simulink model "forcesimulationmodel"  (R2023a)
settings: Solver=VariableStepAuto  StartTime=0.0  StopTime=0.06  RelTol=1e-3
undefined symbols (not defined in the file): tstep
settings Model: Creator=s202421  LastModifiedBy=s202421

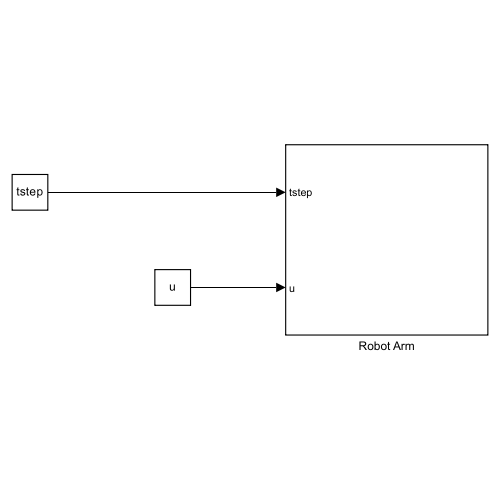
[thumbnail: Simulink's stored preview of the top-level diagram]
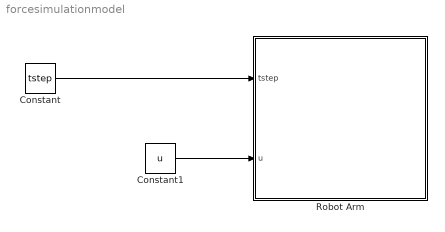
== system forcesimulationmodel ==
  Constant : Constant  Value=tstep
  Constant1 : Constant  Value=u
  Robot Arm : Subsystem
  wires:
  Constant/1 -> Robot Arm/1(tstep)
  Constant1/1 -> Robot Arm/2(u)

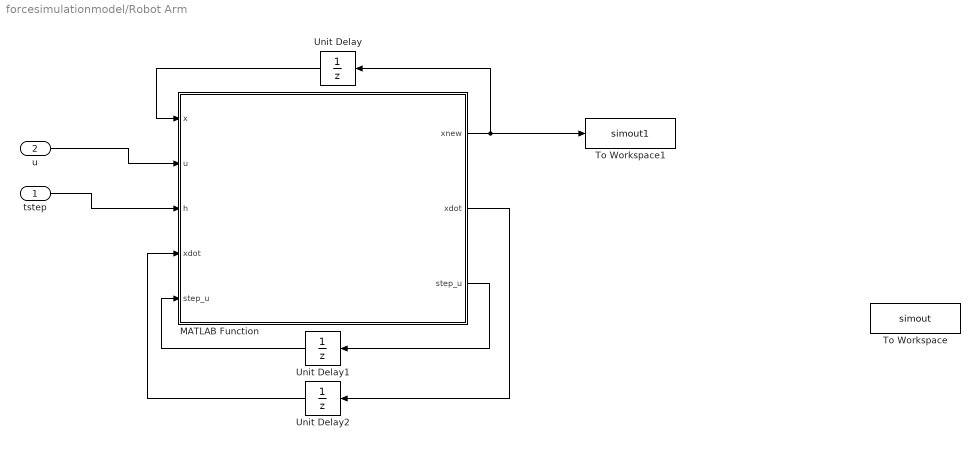
== system forcesimulationmodel/Robot Arm ==
  tstep : Inport
  u : Inport  Port=2
  MATLAB Function : MATLAB Function  TreatAsAtomicUnit=on
  To Workspace : ToWorkspace  VariableName=simout  SaveFormat=Timeseries  SampleTime=-1
  To Workspace1 : ToWorkspace  VariableName=simout1  SaveFormat=Timeseries  SampleTime=-1
  Unit Delay : UnitDelay  SampleTime=-1  HasFrameUpgradeWarning=on
  Unit Delay1 : UnitDelay  SampleTime=-1  HasFrameUpgradeWarning=on
  Unit Delay2 : UnitDelay  SampleTime=-1  HasFrameUpgradeWarning=on
  wires:
  MATLAB Function/1(xnew) -> Unit Delay/1, To Workspace1/1
  ? -> To Workspace/1
  MATLAB Function/2(xdot) -> Unit Delay2/1
  MATLAB Function/3(step_u) -> Unit Delay1/1
  tstep/1 -> MATLAB Function/3(h)
  u/1 -> MATLAB Function/2(u)
  Unit Delay/1 -> MATLAB Function/1(x)
  Unit Delay1/1 -> MATLAB Function/5("step_u ")
  Unit Delay2/1 -> MATLAB Function/4("xdot ")

== matlab function forcesimulationmodel/Robot Arm/MATLAB Function ==
  data: xnew output size=[298 1]; x input size=[298 1]; u input size=[138 1]; h input; xdot input size=[298 1]; xdot output size=[298 1]; step_u output size=[138 1]; step_u input size=[138 1]
function [xnew, xdot, step_u]  = das3step(x, u, h, xdot, step_u)
    coder.extrinsic("das3")
    xnew = zeros(298,1);
    dfdx = ones(298,298);
    dfdxdot=ones(298,298);
    dfdu = ones(298,138);
    f = zeros(298,1);

	% Ton van den Bogert
	% (c) 2010-2011 Case Western Reserve University
    %
	% For dynamic simulation.  Advances the model by one time step.
    %
	% Inputs
	%	x		(298 x 1) System state
	%	u		(138 x 1) Muscle excitations, assumed constant during the time step
	%	h		(scalar)  Time step size
    %   xdot    (298 x 1) System state derivatives (initially zero)
	%	step_u	(138 x 1) Muscle excitations from previous step (initially zero)
    %
    % Optional inputs
    % 	M		(5 x 1)	  Moments applied to the thorax-humerus YZY axes and the elbow flexion and supination axes
	%   exF     (2 x 1)   Vertical force of amplitude exF(2) applied to the ulna at a distance of exF(1) from the elbow 
	%						(to simulate a mobile arm support)
    %   handF   (3 x 1)   Force at the CoM of the hand
    %
	% Outputs
	%	xnew	(298 x 1) The system state at the end of the time step
	%	FGH		(3 x 1)   The glenohumeral reaction force, acting on the scapula
    %
	% Method: First order Rosenbrock formula on implicit differential equation	
	
	% Evaluate dynamics in current x and xdot
    if nargin>7
        [f, dfdx, dfdxdot, dfdu, FGH] = das3('Dynamics',x,xdot,step_u,M,exF,handF);
    elseif nargin>6
        [f, dfdx, dfdxdot, dfdu, FGH] = das3('Dynamics',x,xdot,step_u,M,exF);
    elseif nargin>5
        [f, dfdx, dfdxdot, dfdu, FGH] = das3('Dynamics',x,xdot,step_u,M);
    else
        das3('Dynamics',x,xdot,step_u);
    end
    
	% Solve the change in x from the 1st order Rosenbrock formula
	du = u - step_u;
	dx = (dfdx + dfdxdot/h)\(dfdxdot*xdot - f - dfdu*du);
	xnew = x + dx;
	
	% update variables for the next simulation step
	xdot = dx/h;
	step_u = u;
